simulink model "thermostat_demo"  (R2021a)
settings: Solver=VariableStepAuto  StartTime=0.0  StopTime=30  MaxStep=0.01  RelTol=1e-4  EnableMultiTasking=on
PreLoadFcn:
  | run("thermal_data.m");
  | run("pid_1.m");
model workspace (MAT data in the model file):
  desired_temp = 30
undefined symbols (not defined in the file): c, integral, M, Mdot, proportional, Req, TinIC
settings Model: Creator=llemke  LastModifiedBy=llemke
settings SolverCC: AlgebraicLoopSolver=TrustRegion
settings DataIOCC: LimitDataPoints=on  SaveOutput=off  SaveTime=off
settings OptimizationCC: ExpressionDepthLimit=2147483647  LifeSpan=1
settings DebuggingCC: UnderspecifiedInitializationDetection=Classic  MergeDetectMultiDrivingBlocksExec=none  FcnCallInpInsideContextMsg=warning  AllowSymbolicDim=off  StateNameClashWarn=warning  SFUnexpectedBacktrackingDiag=warning  SFNoUnconditionalDefaultTransitionDiag=warning  SFExecutionAtInitializationDiag=none  SFMachineParentedDataDiag=warning  ArithmeticOperatorsInVariantConditions=warning
settings SFSimCC: SimUseLocalCustomCode=off  CustomCodeUndefinedFunction=UseInterfaceOnly
settings RTWCC: RTWUseLocalCustomCode=off
settings CodeAppCC: StateflowObjectComments=on
settings GRTTargetCC: TargetLangStandard=C89/C90 (ANSI)  CombineOutputUpdateFcns=off  GRTInterface=on

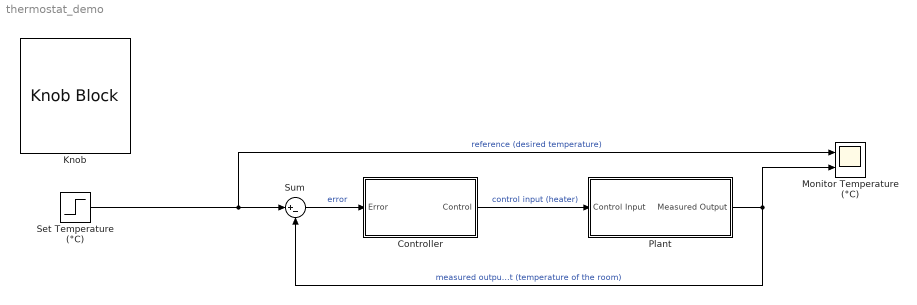
== system thermostat_demo ==
  Controller : Subsystem
  Knob : KnobBlock
  Monitor Temperature (°C) : Scope  NumInputPorts=2
  Plant : Subsystem
  Set Temperature (°C) : Step  Time=5  After=30  SampleTime=0
  Sum : Sum  Inputs=|+-
  wires:
  Set Temperature (°C)/1 -> Sum/1, Monitor Temperature (°C)/1  "reference (desired temperature)"
  Plant/1(Measured Output) -> Monitor Temperature (°C)/2, Sum/2  "measured output (temperature of the room)"
  Sum/1 -> Controller/1(Error)  "error"
  Controller/1(Control) -> Plant/1(Control Input)  "control input (heater)"

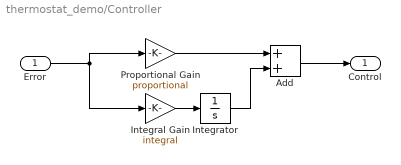
== system thermostat_demo/Controller ==
  Error : Inport
  Add : Sum
  Integral Gain : Gain  Gain=integral
  Integrator : Integrator
  Proportional Gain : Gain  Gain=proportional
  Control : Outport
  wires:
  Error/1 -> Integral Gain/1, Proportional Gain/1
  Add/1 -> Control/1
  Integral Gain/1 -> Integrator/1
  Proportional Gain/1 -> Add/1
  Integrator/1 -> Add/2

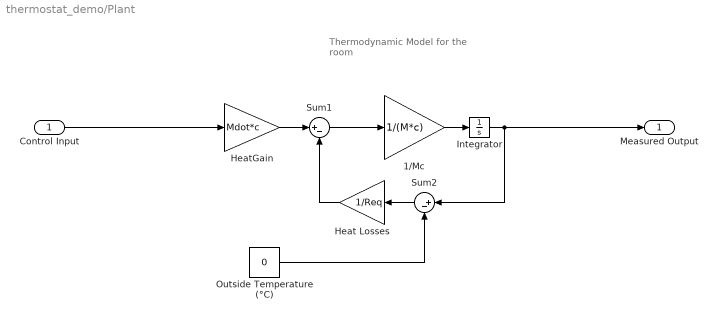
== system thermostat_demo/Plant ==
  note: Thermodynamic Model
      | for the room
  Control Input : Inport
  1/Mc : Gain  Gain=1/(M*c)  SaturateOnIntegerOverflow=on  OutDataTypeStr=Inherit: Same as input  ParamDataTypeStr=Inherit: Same as input
  Heat Losses : Gain  Gain=1/Req  SaturateOnIntegerOverflow=on  OutDataTypeStr=Inherit: Same as input  ParamDataTypeStr=Inherit: Same as input
  HeatGain : Gain  Gain=Mdot*c
  Integrator : Integrator  InitialCondition=TinIC
  Outside Temperature (°C) : Constant  Value=0
  Sum1 : Sum  Inputs=|+-  InputSameDT=on  SaturateOnIntegerOverflow=on  OutDataTypeStr=Inherit: Same as first input
  Sum2 : Sum  Inputs=|+-  InputSameDT=on  SaturateOnIntegerOverflow=on  OutDataTypeStr=Inherit: Same as first input
  Measured Output : Outport
  wires:
  Control Input/1 -> HeatGain/1
  Sum1/1 -> 1/Mc/1
  Outside Temperature (°C)/1 -> Sum2/2
  Integrator/1 -> Measured Output/1, Sum2/1
  Sum2/1 -> Heat Losses/1
  1/Mc/1 -> Integrator/1
  Heat Losses/1 -> Sum1/2
  HeatGain/1 -> Sum1/1
